simulink model "lookup_nD_TestGen40"  (R2017b)
settings: Solver=FixedStepDiscrete  StartTime=0.0  StopTime=10.0  RelTol=1e-3
settings Model: Creator=ktrinh  LastModifiedBy=ktrinh
settings DebuggingCC: ParameterOverflowMsg=none

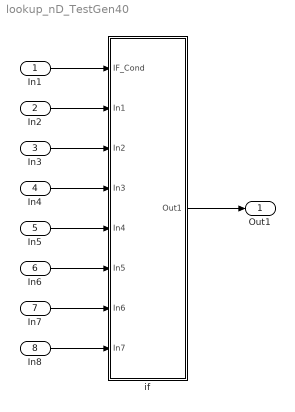
== system lookup_nD_TestGen40 ==
  In1 : Inport
  In2 : Inport  Port=2
  In3 : Inport  Port=3
  In4 : Inport  Port=4
  In5 : Inport  Port=5
  In6 : Inport  Port=6
  In7 : Inport  Port=7
  In8 : Inport  Port=8
  if : Subsystem  AncestorBlock=Block_TestLib/if
  Out1 : Outport
  wires:
  In1/1 -> if/1(IF_Cond)
  In2/1 -> if/2(In1)
  In3/1 -> if/3(In2)
  In4/1 -> if/4(In3)
  In5/1 -> if/5(In4)
  In6/1 -> if/6(In5)
  In7/1 -> if/7(In6)
  In8/1 -> if/8(In7)
  if/1(Out1) -> Out1/1

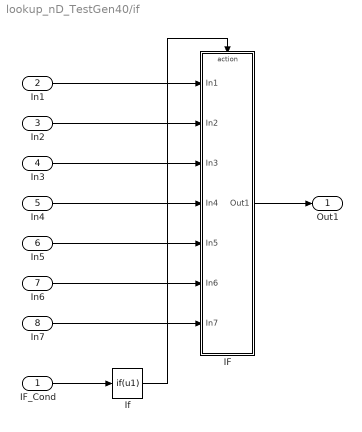
== system lookup_nD_TestGen40/if ==
  IF_Cond : Inport  OutDataTypeStr=boolean
  In1 : Inport  Port=2
  In2 : Inport  Port=3
  In3 : Inport  Port=4
  In4 : Inport  Port=5
  In5 : Inport  Port=6
  In6 : Inport  Port=7
  In7 : Inport  Port=8
  IF : Subsystem  TreatAsAtomicUnit=on
  If : If  IfExpression=u1  ShowElse=off
  Out1 : Outport
  wires:
  If/1 -> IF/Action
  In1/1 -> IF/1(In1)
  In2/1 -> IF/2(In2)
  In3/1 -> IF/3(In3)
  In4/1 -> IF/4(In4)
  In5/1 -> IF/5(In5)
  In6/1 -> IF/6(In6)
  In7/1 -> IF/7(In7)
  IF_Cond/1 -> If/1
  IF/1(Out1) -> Out1/1

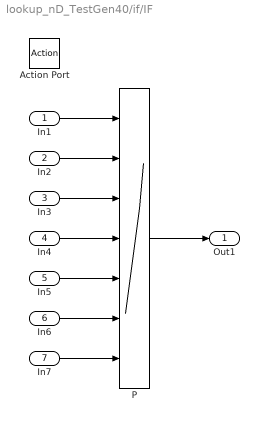
== system lookup_nD_TestGen40/if/IF ==
  In1 : Inport  OutMin=0  OutMax=127  PortDimensions=3
  In2 : Inport  Port=2  OutMin=0  OutMax=127
  In3 : Inport  Port=3  OutMin=0  OutMax=127
  In4 : Inport  Port=4  OutMin=0  OutMax=127
  In5 : Inport  Port=5  OutMin=0  OutMax=127
  In6 : Inport  Port=6  OutMin=0  OutMax=127
  In7 : Inport  Port=7  OutMin=0  OutMax=127
  Action Port : ActionPort  ActionType=then
  P : Lookup_n-D  NumberOfTableDimensions=7  BreakpointsSpecification=Even spacing  BreakpointsForDimension3=[5, 7]  BreakpointsForDimension1FirstPoint=125.4554  BreakpointsForDimension2FirstPoint=58.6595  BreakpointsForDimension3FirstPoint=97.2708  BreakpointsForDimension4FirstPoint=94.9059  BreakpointsForDimension5FirstPoint=59.6941  BreakpointsForDimension6FirstPoint=56.9264  BreakpointsForDimension7FirstPoint=102.0808  BreakpointsForDimension1Spacing=1.5  BreakpointsForDimension2Spacing=1.5  BreakpointsForDimension3Spacing=1.5  BreakpointsForDimension4Spacing=1.5  BreakpointsForDimension5Spacing=1.5  BreakpointsForDimension6Spacing=1.5  BreakpointsForDimension7Spacing=1.5  Table=reshape(repmat([4 5 6 7 8;16 19 20 21 22;10 18 23 24 25],18,8),[2,5,3,2,3,4,3])  InterpMethod=Nearest  UseLastTableValue=on  InternalRulePriority=Speed  RndMeth=Simplest  InputSameDT=on
  Out1 : Outport
  wires:
  In1/1 -> P/1
  In2/1 -> P/2
  In3/1 -> P/3
  In4/1 -> P/4
  In5/1 -> P/5
  In6/1 -> P/6
  In7/1 -> P/7
  P/1 -> Out1/1
